simulink model "z5_dir_2"  (R2015a)
settings: Solver=FixedStepDiscrete  StartTime=0.0  StopTime=99.0  FixedStep=1  RelTol=1e-3
settings Model: Creator=Bojana Vasic  LastModifiedBy=Bojana Vasic

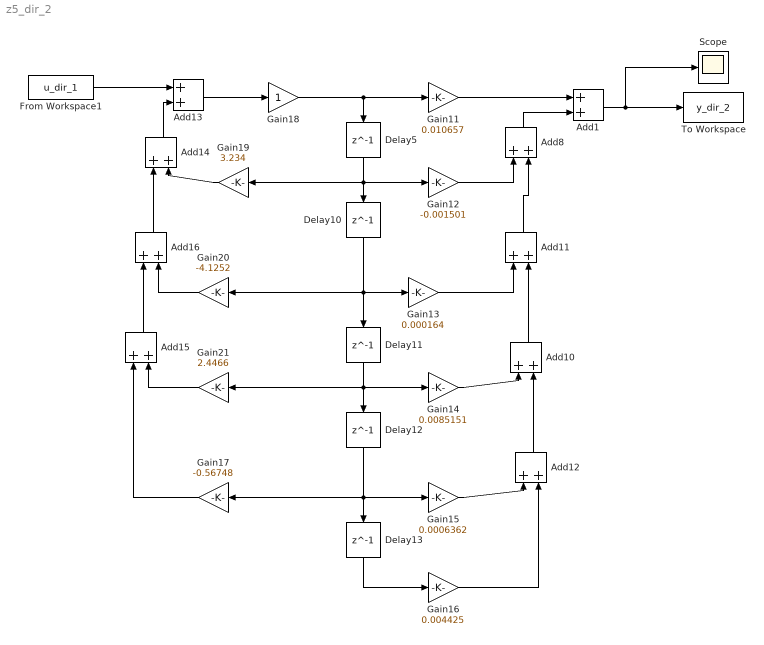
== system z5_dir_2 ==
  Add{1,8,10..16} (9 alike) : Sum
  Delay{5,10..13} (5 alike) : Delay  DelayLength=1
  From Workspace1 : FromWorkspace  VariableName=u_dir_1  SampleTime=1
  Gain11 : Gain  Gain=0.010657
  Gain12 : Gain  Gain=-0.001501
  Gain13 : Gain  Gain=0.000164
  Gain14 : Gain  Gain=0.0085151
  Gain15 : Gain  Gain=0.0006362
  Gain16 : Gain  Gain=0.004425
  Gain17 : Gain  Gain=-0.56748
  Gain18 : Gain
  Gain19 : Gain  Gain=3.234
  Gain20 : Gain  Gain=-4.1252
  Gain21 : Gain  Gain=2.4466
  Scope : Scope
  To Workspace : ToWorkspace  VariableName=y_dir_2  SampleTime=-1
      settings: Save2DSignal=2-D array (concatenate along first dimension)
  wires:
  Gain18/1 -> Gain11/1, Delay5/1
  Gain12/1 -> Add8/1
  Add11/1 -> Add8/2
  Delay10/1 -> Gain13/1, Delay11/1, Gain20/1
  Delay11/1 -> Delay12/1, Gain21/1, Gain14/1
  Gain14/1 -> Add10/1
  Gain13/1 -> Add11/1
  Add10/1 -> Add11/2
  Delay12/1 -> Gain15/1, Delay13/1, Gain17/1
  Delay13/1 -> Gain16/1
  Add12/1 -> Add10/2
  Gain15/1 -> Add12/1
  Gain16/1 -> Add12/2
  Add13/1 -> Gain18/1
  Gain19/1 -> Add14/2
  Add14/1 -> Add13/2
  Add16/1 -> Add14/1
  Gain20/1 -> Add16/2
  Gain21/1 -> Add15/2
  Add15/1 -> Add16/1
  Gain17/1 -> Add15/1
  From Workspace1/1 -> Add13/1
  Delay5/1 -> Gain12/1, Gain19/1, Delay10/1
  Add8/1 -> Add1/2
  Gain11/1 -> Add1/1
  Add1/1 -> Scope/1, To Workspace/1
